simulink model "Ford_T3T6_ArchCnctnDigrm"  (R2016b)
settings: Solver=FixedStepDiscrete  StartTime=0.0  StopTime=10.0  RelTol=1e-3  EnableMultiTasking=on
libraries: canmsglib x15
(part 14 of 15)

== system Ford_T3T6_ArchCnctnDigrm/Ford CFs/FIH Read and Write/FIH write/CF055A_FordBlaBoxCanHiSpdWr1 ==
  EcuId : Inport
  FordEpsSysSt : Inport  Port=2
  FordVehBBMsgOutp1HiPart : Outport
  FordVehBBMsgOutp1LoPart : Outport  Port=2
  FordVehBBMsgOutp2HiPart : Outport  Port=3
  FordVehBBMsgOutp2LoPart : Outport  Port=4
  FordVehBBMsgOutp3HiPart : Outport  Port=5
  FordVehBBMsgOutp3LoPart : Outport  Port=6
  FordVehBBMsgOutp4HiPart : Outport  Port=7
  FordVehBBMsgOutp4LoPart : Outport  Port=8
  FordVehHitchToTrlrAxle : Outport  Port=9
  FordVehLaneAssiAvl : Outport  Port=10
  FordVehLaneAssiDeny : Outport  Port=11
  FordVehLaneAssiHandsOff : Outport  Port=12
  FordVehLatCtrlLimSts : Outport  Port=13
  FordVehLatCtrlSteerSts : Outport  Port=14
  FordVehLoSpdMtnCtrlBrkDecelEnaReq : Outport  Port=15
  FordVehLoSpdMtnCtrlBrkTqReq : Outport  Port=16
  FordVehTrfcJamAvdncHandsOnConf : Outport  Port=17
  FordVehTrlrAgMax : Outport  Port=18
  FordVehTrlrAgOffs : Outport  Port=19
  FordVehTrlrAgTarCalcn : Outport  Port=20
  FordVehTrlrAgWarn : Outport  Port=21
  FordVehTrlrAidEnaSts : Outport  Port=22
  FordVehTrlrAidMsgTxtReq : Outport  Port=23
  FordVehTrlrAidSetupSts : Outport  Port=24
  FordVehTrlrAidTarIdnReq : Outport  Port=25
  FordVehTrlrAidTrlredReq : Outport  Port=26
  FordVehTrlrHitchLampReq : Outport  Port=27
  FordVehVelMaxReqTrlrAid : Outport  Port=28
  FordVehVelTrlrAidReq : Outport  Port=29
  FIH_Write_FIH_Msg_1_High : Outport  Port=30
  FIH_Write_FIH_Msg_1_Low : Outport  Port=31
  FIH_Write_FIH_Msg_2_High : Outport  Port=32
  FIH_Write_FIH_Msg_2_Low : Outport  Port=33
  FIH_Write_FIH_Msg_3_High : Outport  Port=34
  FIH_Write_FIH_Msg_3_Low : Outport  Port=35
  FIH_Write_FIH_Msg_4_High : Outport  Port=36
  FIH_Write_FIH_Msg_4_Low : Outport  Port=37
  FIH_Write_LATCTL_HS_CAN : Outport  Port=38
  FIH_Write_LA_HS_CAN : Outport  Port=39
  FIH_Write_LsmcBrkDecel_Request : Outport  Port=40
  FIH_Write_TBA_to_EPAS_INFO : Outport  Port=41
  FIH_Write_TBA_to_LA_Data3 : Outport  Port=42
  FIH_Write_TBA_to_TrlrAid_Data2 : Outport  Port=43

== system Ford_T3T6_ArchCnctnDigrm/Ford CFs/FIH Read and Write/FIH write/CF058A_FordBlaBoxDiagcWr ==
  ActvNiblCmpIntSts : Outport
  LaneDprtrWarnIntSts : Outport  Port=2
  LaneKeepAssiIntSts : Outport  Port=3
  LatCtrlIntSts : Outport  Port=4
  PullDriftCmpIntSts : Outport  Port=5
  SrvPullDriftCmpAct : Outport  Port=6
  SrvPullDriftCmpRstVal : Outport  Port=7
  TrlrBackupAssiIntSts : Outport  Port=8
  FIH_Write_ANC_Int_Status_DID : Outport  Port=9
  FIH_Write_LATCTL_Int_Status_DID : Outport  Port=10
  FIH_Write_LDW_Int_Status_DID : Outport  Port=11
  FIH_Write_LKA_Int_Status_DID : Outport  Port=12
  FIH_Write_PDC_Actual_DID : Outport  Port=13
  FIH_Write_PDC_Int_Status_DID : Outport  Port=14
  FIH_Write_PDC_Service_DID : Outport  Port=15
  FIH_Write_TBA_Int_Status_DID : Outport  Port=16

== system Ford_T3T6_ArchCnctnDigrm/Ford CFs/FIH Read and Write/FIH write/CF060A_FordBlaBoxFeatStWr1 ==
  FordActvNiblCtrlFeatSt : Outport
  FordActvNiblCtrlSwVers : Outport  Port=2
  FordActvNiblCtrlTqReq : Outport  Port=3
  FordBlaBoxSwVers : Outport  Port=4
  FordLaneAssiSwVers : Outport  Port=5
  FordLaneDprtrWarnFeatSt : Outport  Port=6
  FordLaneDprtrWarnTqReq : Outport  Port=7
  FordLaneKeepAssiFeatSt : Outport  Port=8
  FordLaneKeepAssiTqReq : Outport  Port=9
  FordLatCtrlFeatSt : Outport  Port=10
  FordLatCtrlTqReq : Outport  Port=11
  FordPullDriftCmpFeatSt : Outport  Port=12
  FordPullDriftCmpLrngFeatSt : Outport  Port=13
  FordPullDriftCmpSwVers : Outport  Port=14
  FordPullDriftCmpTqReq : Outport  Port=15
  FordResrchFctSwVers : Outport  Port=16
  FordTrlrBackupAssiSwVers : Outport  Port=17
  FIH_Write_ANC_Arbiter : Outport  Port=18
  FIH_Write_ANC_SW_Version : Outport  Port=19
  FIH_Write_FIH_SW_Version : Outport  Port=20
  FIH_Write_LATCTL_Arbiter : Outport  Port=21
  FIH_Write_LA_SW_Version : Outport  Port=22
  FIH_Write_LDW_Arbiter : Outport  Port=23
  FIH_Write_LKA_Arbiter : Outport  Port=24
  FIH_Write_PDCLearning_Arbiter : Outport  Port=25
  FIH_Write_PDC_Arbiter : Outport  Port=26
  FIH_Write_PDC_SW_Version : Outport  Port=27
  FIH_Write_RF_SW_Version : Outport  Port=28
  FIH_Write_TBA_SW_Version : Outport  Port=29

== system Ford_T3T6_ArchCnctnDigrm/Ford CFs/FIH Read and Write/FIH write/CF090A_FordBlaBoxCanHiSpdWr2 ==
  EcuId : Inport
  FordEpsSysSt : Inport  Port=2
  FordVehEvasSteerAssiSts : Outport
  FIH_Write_ESA_HS_CAN : Outport  Port=2

== system Ford_T3T6_ArchCnctnDigrm/Ford CFs/FIH Read and Write/FIH write/CF091A_FordBlaBoxDiagcWr2 ==
  FordSteerTqDstbcRejctnIntSts : Outport
  FordEvasSteerAssiIntSts : Outport  Port=2
  FordTqSteerCmpActvnCntr : Outport  Port=3
  FordBrkPlsRednActvnCntr : Outport  Port=4
  FIH_Write_STDR_Int_Status_DID : Outport  Port=5
  FIH_Write_ESA_Int_Status_DID : Outport  Port=6
  FIH_Write_TSC_Activation_Cnt : Outport  Port=7
  FIH_Write_BPR_Activation_Cnt : Outport  Port=8

== system Ford_T3T6_ArchCnctnDigrm/Ford CFs/FIH Read and Write/FIH write/CF092A_FordBlaBoxFeatStWr2 ==
  FordSteerTqDstbcRejctnSwVers : Outport  OutMin=[0]  OutMax=[4294967295]  OutDataTypeStr=uint32  Unit=Uls
  FordEvasSteerAssiSwVers : Outport  Port=2  OutMin=[0]  OutMax=[4294967295]  OutDataTypeStr=uint32  Unit=Uls
  FordSteerDstbcRejctnFeatSt : Outport  Port=3  OutMin=[0]  OutMax=[255]  OutDataTypeStr=uint8  Unit=Cnt
  FordEvasSteerAssiFeatSt : Outport  Port=4  OutMin=[0]  OutMax=[255]  OutDataTypeStr=uint8  Unit=Cnt
  FordSteerTqDstbcRejctnTqReq : Outport  Port=5  OutMin=[-32]  OutMax=[31.99]  Unit=HwNwtMtr
  FordEvasSteerAssiTqReq : Outport  Port=6  OutMin=[-64]  OutMax=[63.99]  Unit=HwNwtMtr

== system Ford_T3T6_ArchCnctnDigrm/Ford CFs/FIH Read and Write/FIH write/CF094A_FordBlaBoxNvmWr1 ==
  EcuId : Inport
  FordBlaBoxLaneAssiByte : Outport
  FordBlaBoxPullDriftCmpByte : Outport  Port=2
  FordBlaBoxTrlrBackupByte : Outport  Port=3
  FIH_LA_Write_NV_Byte : Outport  Port=4
  FIH_PDC_Write_NV_Byte : Outport  Port=5
  FIH_TBA_Write_NV_Byte : Outport  Port=6

== system Ford_T3T6_ArchCnctnDigrm/Generate Steering Command/Openloop Steering Command/GenerateSteeringCommand/Assist ==
  note: NM001
  note: NM001
  note: Is being used by GM CF010C. Do we need in ford??
  note: ASIL D
  note: ASIL D
  note: ASIL B
  note: ASIL D Safety Mech
  note: ASIL D
  note: WIR Not being used
  note: WIR Not being used
  note: Is being used by GM CF010C. Do we need in ford??
  note: NM001
  HwTqSwp : Inport
  Ground{,1..3} (4 alike) : Ground
  SF001A_Assi : Subsystem  Tag=1.6.0  Description=The Assist Function applies an appropriate level of motor torque based on handwheel torque andvehicle speed. Its output is modified according to several inputs from other functions. Theseother factors may modify handwheel torque signal, provide blending to alternative calibration tables,or add/subtract values from the calculated assist value.
      settings: AttributesFormatString=Version: %<Tag>
  SF012A_HysCmp : Subsystem  Tag=1.2.1  Description=This function improves steering precision and feel by compensating for physical friction and efficiency losses. Due to the vibratory nature of a vehicle, the calibrations associated with these physical attributes are allowed to vary according to vehicle speed and the magnitude of Wheel Imbalance Rejection function command. The function includes a feature to deal with changing physical system properties over temperature operating range. It also incorporates calibration tables used to modify how the compensation is applied during transitions between operating quadrants and during periods of near-zero handwheel torque. Finally, the function may be disabled for purposes of bench testing.
      settings: AttributesFormatString=Version: %<Tag>
  SF028A_AssiHiFrq : Subsystem  Tag=1.2.1  Description=This function provides a means of compensating for system inertia and road feedback. It is tunable over both vehicle speed and handwheel torque to obtain the desired level of disturbance rejection under various operating conditions. It passes handwheel torque through a high-pass filter and multiplies the resulting signal by a tunable gain factor. The output is known as high-frequency assist and is simply added to the usual assist calculated elsewhere.
      settings: AttributesFormatString=Version: %<Tag>
  SF029A_StabyCmp : Subsystem  Tag=1.3.2  Description=This function provides in-vehicle stability of EPS behavior. To maximize steering feel, the function blends between two different tunings based on vehicle speed and low frequency handwheel torque. Because system gains may get multiplied by various scale factors, either from serial communications or from other software functions, this function provides a second blending feature. This model is designed using the best-known implementation at this time.
      settings: AttributesFormatString=Version: %<Tag>
  SF034B_AssiPahSum : Subsystem  Tag=1.0.1  Description=This function just merges command signals, and is used for vehicle programs that do not need the extra features of the SF034A firewall function.
      settings: AttributesFormatString=Version: %<Tag>
  AssiCmd : Outport
  AssiCmdBas : Outport  Port=2
  tag scope: AssiCmd=global, AssiCmdBas=global, AssiHiFrqCmd=global, HysCmpCmd=global
  wires:
  SF029A_StabyCmp/1(AssiCmd) -> [AssiCmd], AssiCmd/1
  [FltInj_f32] -> SF029A_StabyCmp/6(FltInj_f32)
  SF001A_Assi/1(AssiCmdBas) -> AssiCmdBas/1, SF034B_AssiPahSum/1(AssiCmdBas), [AssiCmdBas]
  SF028A_AssiHiFrq/1(AssiHiFrqCmd) -> SF034B_AssiPahSum/2(AssiHiFrqCmd), [AssiHiFrqCmd]
  [AssiCmdBasSca] -> SF029A_StabyCmp/1(AssiCmdBasSca)
  [VehSpd] -> SF029A_StabyCmp/5(VehSpd)
  SF034B_AssiPahSum/1(AssiCmdSum) -> SF029A_StabyCmp/2(AssiCmdSum)
  Ground/1 -> SF029A_StabyCmp/3(AssiPahLimrActv)
  [AssiCmdBas] -> SF012A_HysCmp/1(AssiCmdBas)
  [AssiMechT] -> SF012A_HysCmp/2(AssiMechT)
  [HwTq] -> SF012A_HysCmp/3(HwTq)
  [HysCmpCmdDi] -> SF012A_HysCmp/4(HysCmpCmdDi)
  [SysFricOffs] -> SF012A_HysCmp/5(SysFricOffs)
  [VehSpd] -> SF012A_HysCmp/6(VehSpd)
  [HwTqOvrl] -> SF012A_HysCmp/8(HwTqOvrl)
  [FltInj_f32] -> SF012A_HysCmp/9(FltInj_f32)
  SF012A_HysCmp/1(HysCmpCmd) -> [HysCmpCmd], SF034B_AssiPahSum/3(HysCmpCmd)
  Ground1/1 -> SF012A_HysCmp/7(WhlImbRejctnAmp)
  [AssiCmdBasSca] -> SF001A_Assi/1(AssiCmdBasSca)
  [AssiLnrGain] -> SF001A_Assi/2(AssiLnrGain)
  [AssiLnrGainEna] -> SF001A_Assi/3(AssiLnrGainEna)
  HwTqSwp/1 -> SF029A_StabyCmp/4(HwTq), SF028A_AssiHiFrq/1(HwTq), SF001A_Assi/4(HwTq)
  [HwTqHysOvrl] -> SF001A_Assi/5(HwTqHysOvrl)
  [HwTqOvrl] -> SF001A_Assi/6(HwTqOvrl)
  [ThermLimSlowFilMax] -> SF001A_Assi/7(ThermLimSlowFilMax)
  [VehSpd] -> SF001A_Assi/8(VehSpd)
  Ground3/1 -> SF001A_Assi/9(WhlImbRejctnAmp)
  [FltInj_f32] -> SF001A_Assi/10(FltInj_f32)
  [VehSpd] -> SF028A_AssiHiFrq/2(VehSpd)
  Ground2/1 -> SF028A_AssiHiFrq/3(WhlImbRejctnAmp)

== system Ford_T3T6_ArchCnctnDigrm/Generate Steering Command/Openloop Steering Command/GenerateSteeringCommand/Damping ==
  note: NM001
  note: NM001
  note: GM CF:CF025
      | Do we need it in Ford
  note: ASIL D
  note: ASIL D
  note: ASIL D
  note: CMS ?
  note: CMS?
  AssiCmdBas : Inport
  HwTqSwp : Inport  Port=2
  Ground : Ground
  SF003A_Dampg : Subsystem  Tag=1.5.0  Description=This function computes a motor damping torque derived primarily from handwheel velocity and scaled by other factors such as temperature and handwheel torque. Dampg shall be comprised of the sum of motor velocity damping and hydraulic power steering damping. Dampg shall be calibratable based on vehicle speed, handwheel torque, motor velocity, and assist.
      settings: AttributesFormatString=Version: %<Tag>
  SF014A_InertiaCmpVel : Subsystem  Tag=1.14.0  Description="Provide compensation that is dependent on filtering of motor velocity.  Primary purpose is to compensate for motor inertia at low frequencies (inertia compensation) and provide damping acting at higher frequencies (frequency dependent damping)."
      settings: AttributesFormatString=Version: %<Tag>
  SF035B_DampgPahSum : Subsystem  Tag=1.0.1  Description=This function is used for programs that do not need the extra features of the SF35A function.
      settings: AttributesFormatString=Version: %<Tag>
  DampgCmd : Outport
  tag scope: DampgCmdBas=global
  wires:
  SF003A_Dampg/1(DampgCmdBas) -> SF035B_DampgPahSum/1(DampgCmdBas), [DampgCmdBas]
  SF035B_DampgPahSum/1(DampgCmd) -> DampgCmd/1
  SF014A_InertiaCmpVel/1(InertiaCmpVelCmd) -> SF035B_DampgPahSum/2(InertiaCmpVelCmd)
  [InertiaCmpVelCmdDi] -> SF014A_InertiaCmpVel/4(InertiaCmpVelCmdDi)
  [FltInj_f32] -> SF014A_InertiaCmpVel/9(FltInj_f32)
  [VehLgtA] -> SF014A_InertiaCmpVel/6(VehLgtA)
  [InertiaCmpDecelGainDi] -> SF014A_InertiaCmpVel/3(InertiaCmpDecelGainDi)
  [MotVelCrf] -> SF014A_InertiaCmpVel/5(MotVelCrf)
  [VehSpd] -> SF014A_InertiaCmpVel/7(VehSpd)
  Ground/1 -> SF014A_InertiaCmpVel/8(WhlImbRejctnAmp)
  AssiCmdBas/1 -> SF003A_Dampg/1(AssiCmdBas), SF014A_InertiaCmpVel/1(AssiCmdBas)
  [AssiMechT] -> SF003A_Dampg/2(AssiMechT)
  [DampgCmdBasDi] -> SF003A_Dampg/3(DampgCmdBasDi)
  [DampgCmdOvrl] -> SF003A_Dampg/4(DampgCmdOvrl)
  [DampgCmdSca] -> SF003A_Dampg/5(DampgCmdSca)
  HwTqSwp/1 -> SF003A_Dampg/6(HwTq), SF014A_InertiaCmpVel/2(HwTq)
  [MotVelCrf] -> SF003A_Dampg/7(MotVelCrf)
  [VehSpd] -> SF003A_Dampg/8(VehSpd)
  [FltInj_f32] -> SF003A_Dampg/9(FltInj_f32)

== system Ford_T3T6_ArchCnctnDigrm/Generate Steering Command/Openloop Steering Command/GenerateSteeringCommand/Return ==
  note: ASIL B
  note: ASIL D
  note: CMS?
  note: CMS?
  note: CMS?
  note: CMS?
  note: CMS?
  note: NM001
  note: NM001
  note: NM001
  HwTqSwp : Inport
  SF002A_Rtn : Subsystem  Tag=2.3.0  Description="The Return function shall provide return to center capability to enhance vehicle returnability. This is achieved by applying output force toward center as a function of output position and vehicle speed Thisposition-based output is modified for the given driving situation basedon Handwheel  Torque, Handwheel Velocity, and system temperature.Outputcan be defeated or reduced until Handwheel Position is known with fullconfidence, which may occur at startup or upon completion of a learningprocedure. Finally, output is directly scaled higher or lower byadditional inputs (e.g. customer signals, diagnostics)."
      settings: AttributesFormatString=Version: %<Tag>
  SF036A_RtnPahFwl : Subsystem  Tag=1.2.0  Description=This function bounds motor torque commands from SF-02 Active Return, whose primary input is handwheel position. The incoming motor torque command is saturated to a set of upper and lower boundaries chosen according to handwheel position.
      settings: AttributesFormatString=Version: %<Tag>
  RtnCmd : Outport
  tag scope: RtnCmd=global, RtnCmdLimd=global
  wires:
  SF036A_RtnPahFwl/1(RtnCmdLimd) -> RtnCmd/1, [RtnCmdLimd]
  [AssiMechT] -> SF002A_Rtn/1(AssiMechT)
  [HwAg] -> SF002A_Rtn/2(HwAg)
  [HwAgAuthySca] -> SF002A_Rtn/3(HwAgAuthySca)
  [HwAgRtnOffs] -> SF002A_Rtn/4(HwAgRtnOffs)
  HwTqSwp/1 -> SF002A_Rtn/5(HwTq)
  [HwVel] -> SF002A_Rtn/6(HwVel)
  [RtnCmdDi] -> SF002A_Rtn/7(RtnCmdDi)
  [RtnCmdDiagcDi] -> SF002A_Rtn/8(RtnCmdDiagcDi)
  [RtnCmdSca] -> SF002A_Rtn/9(RtnCmdSca)
  [RtnCmdScaServo] -> SF002A_Rtn/10(RtnCmdScaServo)
  [VehSpd] -> SF002A_Rtn/11(VehSpd)
  [VehSpdVld] -> SF002A_Rtn/12(VehSpdVld)
  [FltInj_f32] -> SF002A_Rtn/13(FltInj_f32)
  [HwAg] -> SF036A_RtnPahFwl/1(HwAg)
  [MfgEnaSt] -> SF036A_RtnPahFwl/2(MfgEnaSt)
  SF002A_Rtn/1(RtnCmd) -> [RtnCmd]
  [RtnCmdDi] -> SF036A_RtnPahFwl/4(RtnCmdDi)
  [VehSpd] -> SF036A_RtnPahFwl/5(VehSpd)
  [SetNtcSts10] -> SF036A_RtnPahFwl/6(SetNtcSts)
  [RtnCmd] -> SF036A_RtnPahFwl/3(RtnCmd)

== system Ford_T3T6_ArchCnctnDigrm/Generate Steering Command/Openloop Steering Command/GenerateSteeringCommand/SF004B_AssiSumLim ==
  AssiCmd : Inport
  DampgCmd : Inport  Port=2
  EotActvCmd : Inport  Port=3
  EotAssiSca : Inport  Port=4
  EotDampgCmd : Inport  Port=5
  EotMotTqLim : Inport  Port=6
  HwTqLoaMtgtnEna : Inport  Port=7
  MotTqCmdLimDi : Inport  Port=8
  MotTqCmdOvrl : Inport  Port=9
  MotVelMrf : Inport  Port=10
  PinionCentrLrnCmd : Inport  Port=11
  PinionCentrLrnEna : Inport  Port=12
  PullCmpCmd : Inport  Port=13
  PwrLimrRednFac : Inport  Port=14
  RtnCmd : Inport  Port=15
  StallMotTqLim : Inport  Port=16
  SysMotTqCmdSca : Inport  Port=17
  ThermMotTqLim : Inport  Port=18
  ThermRednFac : Inport  Port=19
  TqLoaCmd : Inport  Port=20
  TqSteerMtgtnCmd : Inport  Port=21
  VehSpd : Inport  Port=22
  VehSpdMotTqLim : Inport  Port=23
  WhlImbRejctnCmd : Inport  Port=24
  GetNtcQlfrSts : Inport  Port=25
  SetNtcSts : Inport  Port=26
  MotTqCmd : Outport
  MotTqCmdLimdPreStall : Outport  Port=2
  MotTqCmdLimrMin : Outport  Port=3
  MotTqCmdPreLim : Outport  Port=4
  SysProtnRednFac : Outport  Port=5
  SetManTqCmd : Outport  Port=6

== system Ford_T3T6_ArchCnctnDigrm/Generate Steering Command/Openloop Steering Command/GenerateSteeringCommand/SF020B_PosnTrakgServo ==
  HwAg : Inport
  HwTq : Inport  Port=2
  MotVelCrf : Inport  Port=3
  PosnServoEna : Inport  Port=4
  PosnServoHwAg : Inport  Port=5
  PosnServoHwVel : Inport  Port=6
  PosnServoIntgtrOffs : Inport  Port=7
  PosnTrakgArbnFltMtgtnEna : Inport  Port=8
  VehSpd : Inport  Port=9
  PosnServoCmd : Outport
  PosnServoIntgtrSt : Outport  Port=2

== system Ford_T3T6_ArchCnctnDigrm/Generate Steering Command/Openloop Steering Command/System Protection/EoTProtection ==
  note: ASIL B
  note: ASIL B
  note: ASIL D
  note: NM001
  note: NM001
  note: NM001
  SF016A_VehSpdLimr : Subsystem  Tag=2.0.1  Description=The Vehicle Speed Limiting Function determines a limited assist torque command value as a function of vehicle speed and handwheel position to manage mechanical fatigue near end-of-travel positions.
      settings: AttributesFormatString=Version: %<Tag>
  SF018A_EotProtn : Subsystem  Tag=1.11.0  Description=The End of Travel Protection function specifies performance attributes as the steering system approaches the mechanical end of travel of the steering gear. There are three primary functions: Velocity Impact (VI), Soft Stops (SS), and Software Rack Limiter (SRL). The purpose of VI is to limit the assist for high steering velocity. The purpose of SS is to scale down the assist and provide damping. The SRL is intended to simulate a hardware rack limiter.
      settings: AttributesFormatString=Version: %<Tag>
  SF027A_EotProtnFwl : Subsystem  Tag=1.3.1  Description="This function applies boundary limitations on motor torque commands from SF018A (EOT Protection)including the EOTDamping and EOTActive.   The motor torque commands are saturation limited toupper and lower boundaries.  Three criteria are tested to determine the firewall limit to be applied:1) Determine if a command is within a statically dterined intended active range for the EOT Protectionfunction.  This contrasts with the dynamically determined active range for SF018 based on the learnedend of travel limits.  If determined to be within the active range then apply an upper and lower boundary.2) If Handwheel Position is inboard of the active region (eg between +/- X0) then apply simple saturationlimit preventing a large command from being output.3) If Handwheel Authority is below a  calibration threshold value, then apply a simple saturation limitpreventing a large command from being output."
      settings: AttributesFormatString=Version: %<Tag>
  EotActvCmd : Outport
  EotDampgCmd : Outport  Port=2
  EotAssiSca : Outport  Port=3
  EotMotTqLim : Outport  Port=4
  VehSpdMotTqLim : Outport  Port=5
  tag scope: EotActvCmd=global, EotAssiSca=global, EotDampgCmd=global, EotMotTqLim=global
  wires:
  SF018A_EotProtn/2(EotAssiSca) -> EotAssiSca/1, [EotAssiSca]
  SF018A_EotProtn/4(EotMotTqLim) -> EotMotTqLim/1, [EotMotTqLim]
  [HwAg] -> SF016A_VehSpdLimr/1(HwAg)
  [PinionAgConf] -> SF016A_VehSpdLimr/2(HwAgAuthy)
  [HwAgEotCcw] -> SF016A_VehSpdLimr/3(HwAgEotCcw)
  [HwAgEotCw] -> SF016A_VehSpdLimr/4(HwAgEotCw)
  [VehSpd] -> SF016A_VehSpdLimr/5(VehSpd)
  SF016A_VehSpdLimr/1(VehSpdMotTqLim) -> VehSpdMotTqLim/1
  [EotProtnDi] -> SF027A_EotProtnFwl/3(EotProtnDi)
  [HwAg] -> SF027A_EotProtnFwl/4(HwAg)
  [MfgEnaSt] -> SF027A_EotProtnFwl/5(MfgEnaSt)
  [MotVelCrf] -> SF027A_EotProtnFwl/6(MotVelCrf)
  [PinionAgConf] -> SF027A_EotProtnFwl/7(PinionAgConf)
  [VehSpd] -> SF027A_EotProtnFwl/8(VehSpd)
  [SetNtcSts] -> SF027A_EotProtnFwl/9(SetNtcSts)
  SF018A_EotProtn/1(EotActvCmd) -> SF027A_EotProtnFwl/1(EotActvCmd), [EotActvCmd]
  SF018A_EotProtn/3(EotDampgCmd) -> SF027A_EotProtnFwl/2(EotDampgCmd), [EotDampgCmd]
  SF027A_EotProtnFwl/1(EotActvCmdLimd) -> EotActvCmd/1
  SF027A_EotProtnFwl/2(EotDampgCmdLimd) -> EotDampgCmd/1
  [EotProtnDi] -> SF018A_EotProtn/1(EotProtnDi)
  [HwAg] -> SF018A_EotProtn/2(HwAg)
  [PinionAgConf] -> SF018A_EotProtn/3(HwAgAuthy)
  [HwAgCcwDetd] -> SF018A_EotProtn/4(HwAgCcwDetd)
  [HwAgCwDetd] -> SF018A_EotProtn/5(HwAgCwDetd)
  [HwAgEotCcw] -> SF018A_EotProtn/6(HwAgEotCcw)
  [HwAgEotCw] -> SF018A_EotProtn/7(HwAgEotCw)
  [HwTq] -> SF018A_EotProtn/8(HwTq)
  [MotVelCrf] -> SF018A_EotProtn/9(MotVelCrf)
  [SysMotTqCmdSca] -> SF018A_EotProtn/10(SysMotTqCmdSca)
  [VehSpd] -> SF018A_EotProtn/11(VehSpd)

== system Ford_T3T6_ArchCnctnDigrm/Generate Steering Command/Openloop Steering Command/System Protection/Motor Protection ==
  note: Which MM??
  note: ASIL B
  note: ASIL B
  note: Which MM??
  note: NM001
  note: NM001
  MotTqCmdLimdPreStall : Inport
  SF009A_DutyCycThermProtn : Subsystem  Tag=4.0.0  Description=The purpose of the Thermal Duty Cycle Protection is to limitand protect the system from excessive use, based on motor rotational velocity and system temperature.It also provides protection status information for use by other functions.
      settings: AttributesFormatString=Version: %<Tag>
  SF017A_HiLoadStallLimr : Subsystem  Tag=3.0.0  Description="This function protects the system from prolonged intervals of high assist torque at near-stall conditions.  In other words, it quickly limits large torque commands if the motor velocity is below a calibratable threshold. The High Load Stall Limiter function uses a low-pass filter (LPF) and a torque limit table to reduce the maximum allowed torque command under certain operating conditions.  When motor velocity is equal to or falls below the calibratable threshold, the torque command is applied to the input of the low-pass filter.  The output of the filter ramps up and indexes into the torque limit table.  The output of this table is the maximum allowed torque command.  A slew limit calibration governs the transition rate of the table output."
      settings: AttributesFormatString=Version: %<Tag>
  StallMotTqLim : Outport
  ThermMotTqLim : Outport  Port=2
  tag scope: DutyCycThermProtnMaxOutp=global, StallMotTqLim=global, ThermDutyCycProtnLoadDptLim=global, ThermDutyCycProtnTDptLim=global, ThermLimSlowFilMax=global, ThermMotTqLim=global, ThermRednFac=global
  wires:
  SF009A_DutyCycThermProtn/5(ThermMotTqLim) -> ThermMotTqLim/1, [ThermMotTqLim]
  [DualEcuFltMtgtnEna] -> SF017A_HiLoadStallLimr/1(DualEcuFltMtgtnEna)
  [MotAndThermProtnLoaMod] -> SF017A_HiLoadStallLimr/2(MotAndThermProtnLoaMod)
  MotTqCmdLimdPreStall/1 -> SF017A_HiLoadStallLimr/3(MotTqCmdLimdPreStall)
  [MotVelCrf] -> SF017A_HiLoadStallLimr/4(MotVelCrf)
  [StallMotTqLimDi] -> SF017A_HiLoadStallLimr/5(StallMotTqLimDi)
  SF017A_HiLoadStallLimr/1(StallMotTqLim) -> StallMotTqLim/1, [StallMotTqLim]
  [DiagcStsLimdTPrfmnc] -> SF009A_DutyCycThermProtn/1(DiagcStsLimdTPrfmnc)
  [DualEcuFltMtgtnEna] -> SF009A_DutyCycThermProtn/2(DualEcuFltMtgtnEna)
  [DutyCycThermProtnDi] -> SF009A_DutyCycThermProtn/3(DutyCycThermProtnDi)
  [EcuTFild] -> SF009A_DutyCycThermProtn/4(EcuTFild)
  [IgnTiOff] -> SF009A_DutyCycThermProtn/5(IgnTiOff)
  [MotAndThermProtnLoaMod] -> SF009A_DutyCycThermProtn/6(MotAndThermProtnLoaMod)
  [MotCurrPeakEstimd] -> SF009A_DutyCycThermProtn/7(MotCurrPeakEstimd)
  [MotCurrPeakEstimdFild] -> SF009A_DutyCycThermProtn/8(MotCurrPeakEstimdFild)
  [MotFetT] -> SF009A_DutyCycThermProtn/9(MotFetT)
  [MotMagT] -> SF009A_DutyCycThermProtn/10(MotMagT)
  [MotVelCrf] -> SF009A_DutyCycThermProtn/11(MotVelCrf)
  [MotWidgT] -> SF009A_DutyCycThermProtn/12(MotWidgT)
  [VehTiVld] -> SF009A_DutyCycThermProtn/13(VehTiVld)
  [NvMProxy_GetErrorStatus] -> SF009A_DutyCycThermProtn/14(FilStVal_GetErrorStatus)
  [NvMProxy_SetRamBlockStatus] -> SF009A_DutyCycThermProtn/15(FilStVal_SetRamBlockStatus)
  [SetNtcSts8] -> SF009A_DutyCycThermProtn/16(SetNtcSts)
  SF009A_DutyCycThermProtn/1(DutyCycThermProtnMaxOutp) -> [DutyCycThermProtnMaxOutp]
  SF009A_DutyCycThermProtn/2(ThermDutyCycProtnLoadDptLim) -> [ThermDutyCycProtnLoadDptLim]
  SF009A_DutyCycThermProtn/3(ThermDutyCycProtnTDptLim) -> [ThermDutyCycProtnTDptLim]
  SF009A_DutyCycThermProtn/4(ThermLimSlowFilMax) -> [ThermLimSlowFilMax]
  SF009A_DutyCycThermProtn/6(ThermRednFac) -> [ThermRednFac]

== system Ford_T3T6_ArchCnctnDigrm/Generate Steering Command/Openloop Steering Command/System Protection/SF038A_LimrCdng ==
  EotAssiSca : Inport
  EotMotTqLim : Inport  Port=2
  StallMotTqLim : Inport  Port=3
  SysMotTqCmdSca : Inport  Port=4
  ThermMotTqLim : Inport  Port=5
  VehSpd : Inport  Port=6
  VehSpdMotTqLim : Inport  Port=7
  FltInj_f32 : Inport  Port=8
  EotAssiScaCdnd : Outport
  EotMotTqLimCdnd : Outport  Port=2
  StallMotTqLimCdnd : Outport  Port=3
  SysMotTqCmdScaCdnd : Outport  Port=4
  ThermMotTqLimCdnd : Outport  Port=5
  VehSpdMotTqLimCdnd : Outport  Port=6

== system Ford_T3T6_ArchCnctnDigrm/Monitor System/Inferred Signals/HwAg before IMC/CF075A_FordHwAgArbn ==
  FordVehSteerPinionAgOffs : Inport
  FordVehSteerPinionOffsSts : Inport  Port=2
  FordVehSteerPinionOffsChks : Inport  Port=3
  FordVehSteerPinionOffsCnt : Inport  Port=4
  HwAgFinal : Inport  Port=5
  HwAgNotCorrd : Inport  Port=6
  PinionVel : Inport  Port=7
  PinionVelConf : Inport  Port=8
  FordAbsPrsnt : Inport  Port=9
  FordSteerAgClrFlg : Inport  Port=10
  HwAgIdptSig : Inport  Port=11
  GetRefTmr100MicroSec32bit : Inport  Port=12
  GetTiSpan100MicroSec32bit : Inport  Port=13
  NonAbsOffsVldFlg_GetErrorStatus : Inport  Port=14
  NonAbsOffsVldFlg_SetRamBlockStatus : Inport  Port=15
  NonAbsOffs_GetErrorStatus : Inport  Port=16
  NonAbsOffs_SetRamBlockStatus : Inport  Port=17
  PrevIgnCycVal_GetErrorStatus : Inport  Port=18
  PrevIgnCycVal_SetRamBlockStatus : Inport  Port=19
  SetNtcSts : Inport  Port=20
  FordCmpdHwPosn : Outport
  FordCmpdHwPosnQlyFac : Outport  Port=2
  FordHwVel : Outport  Port=3
  FordHwVelVld : Outport  Port=4
  FordPosnOffsVld : Outport  Port=5
  FordRelHwPosn : Outport  Port=6
  FordRelHwPosnVld : Outport  Port=7

== system Ford_T3T6_ArchCnctnDigrm/Monitor System/Inferred Signals/HwAg before IMC/SF041A_CmplncErr ==
  HwTq : Inport
  MotTqCmdCrf : Inport  Port=2
  CmplncErrMotToPinion : Outport
  CmplncErrPinionToHw : Outport  Port=2

== system Ford_T3T6_ArchCnctnDigrm/Monitor System/Inferred Signals/HwAg before IMC/SF042A_HwAgSnsrls ==
  CmplncErrMotToPinion : Inport
  HwTq : Inport  Port=2
  MotAgCumvAlgndCrf : Inport  Port=3
  MotAgCumvAlgndVld : Inport  Port=4
  MotAgMeclIdptSig : Inport  Port=5
  MotTqCmdCrf : Inport  Port=6
  MotVelCrf : Inport  Port=7
  PinionAg : Inport  Port=8
  PinionAgConf : Inport  Port=9
  VehSpd : Inport  Port=10
  VehSpdVld : Inport  Port=11
  VehYawRate : Inport  Port=12
  VehYawRateVld : Inport  Port=13
  WhlFrqVld : Inport  Port=14
  WhlLeFrq : Inport  Port=15
  WhlRiFrq : Inport  Port=16
  GetNtcQlfrSts : Inport  Port=17
  GetRefTmr100MicroSec32bit : Inport  Port=18
  GetTiSpan100MicroSec32bit : Inport  Port=19
  StordLstPrm_SetRamBlockStatus : Inport  Port=20
  HwAgSnsrls : Outport
  HwAgSnsrlsConf : Outport  Port=2
  FSnsrlsHwCentr : Outport  Port=3
  RstSnsrlsHwCentr : Outport  Port=4

== system Ford_T3T6_ArchCnctnDigrm/Monitor System/Inferred Signals/HwAg before IMC/SF045A_HwAgSysArbn ==
  CmplncErrPinionToHw : Inport
  HwAg : Inport  Port=2
  HwAgCorrd : Inport  Port=3
  HwAgIdptSig : Inport  Port=4
  HwAgSnsrls : Inport  Port=5
  HwAgSnsrlsConf : Inport  Port=6
  HwTq : Inport  Port=7
  MotVelCrf : Inport  Port=8
  MotVelVld : Inport  Port=9
  GetNtcQlfrSts : Inport  Port=10
  FltInj_f32 : Inport  Port=11
  GetRefTmr100MicroSec32bit : Inport  Port=12
  GetTiSpan100MicroSec32bit : Inport  Port=13
  SetNtcSts : Inport  Port=14
  HwAgFinal : Outport
  HwAgNotCorrd : Outport  Port=2
  HwAgToSerlCom : Outport  Port=3
  HwAgVldToSerlCom : Outport  Port=4
  HwVel : Outport  Port=5
  HwVelToSerlCom : Outport  Port=6
  PinionAg : Outport  Port=7
  PinionAgConf : Outport  Port=8
  PinionVel : Outport  Port=9
  PinionVelConf : Outport  Port=10

== system Ford_T3T6_ArchCnctnDigrm/Monitor System/Measured Signals/ADC/CM012A_FordT3McuCfg ==
  Adc0Faild : Inport
  Adc1Faild : Inport  Port=2
  Adc1RawRes : Inport  Port=3
  EcuId : Inport  Port=4
  MotCtrlAdc0RawRes : Inport  Port=5
  GetRefTmr1MicroSec32bit : Inport  Port=6
  GetTiSpan1MicroSec32bit : Inport  Port=7
  Adc1ScanGroup2Ref0 : Outport
  Adc1ScanGroup2Ref1 : Outport  Port=2
  Adc1ScanGroup3Ref0 : Outport  Port=3
  Adc1ScanGroup3Ref1 : Outport  Port=4
  Adc1SelfDiag0 : Outport  Port=5
  Adc1SelfDiag2 : Outport  Port=6
  Adc1SelfDiag4 : Outport  Port=7
  BattRtnCurrAdc : Outport  Port=8
  BattRtnCurrAdcFaild : Outport  Port=9
  BattVltg : Outport  Port=10
  BattVltgAdcFaild : Outport  Port=11
  BattVltgSwd1 : Outport  Port=12
  BattVltgSwd1AdcFaild : Outport  Port=13
  ChrgPmpDiag : Outport  Port=14
  ChrgPmpDiagAdcFaild : Outport  Port=15
  EcuT : Outport  Port=16
  EcuTAdcFaild : Outport  Port=17
  HwAg1SnsrNr : Outport  Port=18
  HwAg1SnsrTyp : Outport  Port=19
  MotAg2Cos : Outport  Port=20
  MotAg2CosAdcFaild : Outport  Port=21
  MotAg2Sin : Outport  Port=22
  MotAg2SinAdcFaild : Outport  Port=23
  MotAg5CosAdcFaild : Outport  Port=24
  MotAg5SinAdcFaild : Outport  Port=25
  MotAg6CosAdcFaild : Outport  Port=26
  MotAg6SinAdcFaild : Outport  Port=27
  MotCurrAdcPeakAAdcFaild : Outport  Port=28
  MotCurrAdcPeakBAdcFaild : Outport  Port=29
  MotCurrAdcPeakCAdcFaild : Outport  Port=30
  MotCurrAdcVlyAAdcFaild : Outport  Port=31
  MotCurrAdcVlyBAdcFaild : Outport  Port=32
  MotCurrAdcVlyCAdcFaild : Outport  Port=33
  MotCurrSnsrOffs1AdcFaild : Outport  Port=34
  PwrDiscnctSwtDiag : Outport  Port=35
  PwrDiscnctSwtDiagAdcFaild : Outport  Port=36
  MotDrvr1IninTestCmpl : Outport  Port=37
  MotCtrlAdc0ScanGroup2Ref0 : Outport  Port=38
  MotCtrlAdc0ScanGroup2Ref1 : Outport  Port=39
  MotCtrlAdc0ScanGroup3Ref0 : Outport  Port=40
  MotCtrlAdc0ScanGroup3Ref1 : Outport  Port=41
  MotCtrlAdc0SelfDiag0 : Outport  Port=42
  MotCtrlAdc0SelfDiag2 : Outport  Port=43
  MotCtrlAdc0SelfDiag4 : Outport  Port=44
  MotCtrlMotAg5Cos : Outport  Port=45
  MotCtrlMotAg5Sin : Outport  Port=46
  MotCtrlMotAg6Cos : Outport  Port=47
  MotCtrlMotAg6Sin : Outport  Port=48
  MotCtrlMotCurrAdcPeakA : Outport  Port=49
  MotCtrlMotCurrAdcPeakB : Outport  Port=50
  MotCtrlMotCurrAdcPeakC : Outport  Port=51
  MotCtrlMotCurrAdcVlyA : Outport  Port=52
  MotCtrlMotCurrAdcVlyB : Outport  Port=53
  MotCtrlMotCurrAdcVlyC : Outport  Port=54
  MotCtrlMotCurrSnsrOffs1 : Outport  Port=55

== system Ford_T3T6_ArchCnctnDigrm/Monitor System/Measured Signals/ADC/ES251A_BattRtnCurr ==
  BattRtnCurrAdc : Inport  OutMin=[0]  OutMax=[5]  OutDataTypeStr=single  Unit=Volt
  BattRtnCurrAdcFaild : Inport  Port=2  OutMin=[0]  OutMax=[1]  OutDataTypeStr=boolean  Unit=Cnt
  SplyCurrEstim : Inport  Port=3  OutMin=[-200]  OutMax=[200]  OutDataTypeStr=single  Unit=Ampr
  SysSt : Inport  Port=4  OutMin=[0]  OutMax=[3]  Unit=Cnt
  MotCtrlBattRtnCurrAdc : Inport  Port=5  OutMin=[0]  OutMax=[5]  OutDataTypeStr=single  Unit=Volt
  CnvSnpshtData_f32 : Inport  Port=6  OutMin=[[]]  OutMax=[[]]
  CnvSnpshtData_u08 : Inport  Port=7  OutMin=[[]]  OutMax=[[]]
  GetNtcQlfrSts : Inport  Port=8  OutMin=[0]  OutMax=[1]
  SetNtcStsAndSnpshtData : Inport  Port=9  OutMin=[0]  OutMax=[1]
  BattRtnCurrAmpr : Outport  OutMin=[-300]  OutMax=[300]  OutDataTypeStr=single  Unit=Ampr
  BattRtnCurrStsQlfr : Outport  Port=2  OutMin=[0]  OutMax=[2]  Unit=Cnt
  MotCtrlBattRtnCurrAmprFastLoop : Outport  Port=3  OutMin=[-300]  OutMax=[300]  OutDataTypeStr=single  Unit=Ampr

== system Ford_T3T6_ArchCnctnDigrm/Monitor System/Measured Signals/BatteryVoltage/ES250B_BattVltg ==
  BattSwdVltgCorrlnSts : Inport
  BattVltg : Inport  Port=2
  BattVltgSwd1 : Inport  Port=3
  BrdgVltg : Outport

== system Ford_T3T6_ArchCnctnDigrm/Monitor System/Measured Signals/BatteryVoltage/ES259B_BattVltgCorrln ==
  BattVltg : Inport
  BattVltgAdcFaild : Inport  Port=2
  BattVltgSwd1 : Inport  Port=3
  BattVltgSwd1AdcFaild : Inport  Port=4
  DiagcStsIvtr1Inactv : Inport  Port=5
  InhbBattVltgDiagc : Inport  Port=6
  StrtUpSt : Inport  Port=7
  SysSt : Inport  Port=8
  GetNtcQlfrSts : Inport  Port=9
  SetNtcSts : Inport  Port=10
  BattSwdVltgCorrlnSts : Outport
  BattVltgCorrlnIdptSig : Outport  Port=2
  DftBrdgVltgActv : Outport  Port=3
  SwdVltgLimd : Outport  Port=4

== system Ford_T3T6_ArchCnctnDigrm/Monitor System/Measured Signals/EcuTemp/ES210A_EcuTMeas ==
  EcuT : Inport
  EcuTAdcFaild : Inport  Port=2
  CnvSnpshtData_f32 : Inport  Port=3
  CnvSnpshtData_logl : Inport  Port=4
  GetNtcActv : Inport  Port=5
  SetNtcStsAndSnpshtData : Inport  Port=6
  DiagcStsLimdTPrfmnc : Outport
  EcuTFild : Outport  Port=2

== system Ford_T3T6_ArchCnctnDigrm/Monitor System/Measured Signals/HwAg Signal Measurement and  Arbitration/CM670A_HwAg1Meas ==
  HwAg1Polarity : Inport
  HwAg1SnsrTyp : Inport  Port=2
  CnvSnpshtData_f32 : Inport  Port=3
  CnvSnpshtData_u08 : Inport  Port=4
  FltInj_u08 : Inport  Port=5
  GetNtcQlfrSts : Inport  Port=6
  GetRefTmr1MicroSec32bit : Inport  Port=7
  GetTiSpan1MicroSec32bit : Inport  Port=8
  HwAg1IfFltLtch_GetErrorStatus : Inport  Port=9
  HwAg1IfFltLtch_SetRamBlockStatus : Inport  Port=10
  HwAg1Offs_GetErrorStatus : Inport  Port=11
  HwAg1Offs_SetRamBlockStatus : Inport  Port=12
  IoHwAb_SetFctPrphlHwAg1 : Inport  Port=13
  SetNtcStsAndSnpshtData : Inport  Port=14
  HwAg1 : Outport
  HwAg1Qlfr : Outport  Port=2
  HwAg1RollgCntr : Outport  Port=3
  HwAg1AutTrim : Outport  Port=4
  HwAg1ClrLtch : Outport  Port=5
  HwAg1ClrTrim : Outport  Port=6
  HwAg1ReadTrim : Outport  Port=7
  HwAg1TrimPrfmdSts : Outport  Port=8
  HwAg1WrTrim : Outport  Port=9

== system Ford_T3T6_ArchCnctnDigrm/Monitor System/Measured Signals/HwAg Signal Measurement and  Arbitration/ES238A_HwAgArbn ==
  HwAg1SnsrNr : Inport  OutMin=[0]  OutMax=[2]  OutDataTypeStr=uint8  Unit=Cnt
  HwAgA : Inport  Port=2  OutMin=[-900]  OutMax=[900]  OutDataTypeStr=single  Unit=HwDeg
  HwAgAQlfr : Inport  Port=3  OutMin=[0]  OutMax=[2]  OutDataTypeStr=Enum: SigQlfr1  Unit=Cnt
  HwAgARollgCntr : Inport  Port=4  OutMin=[0]  OutMax=[255]  OutDataTypeStr=uint8  Unit=Cnt
  HwAgB : Inport  Port=5  OutMin=[-900]  OutMax=[900]  OutDataTypeStr=single  Unit=HwDeg
  HwAgBQlfr : Inport  Port=6  OutMin=[0]  OutMax=[2]  OutDataTypeStr=Enum: SigQlfr1  Unit=Cnt
  HwAgBRollgCntr : Inport  Port=7  OutMin=[0]  OutMax=[255]  OutDataTypeStr=uint8  Unit=Cnt
  HwAgCorrlnSt : Inport  Port=8  OutMin=[0]  OutMax=[3]  OutDataTypeStr=uint8  Unit=Cnt
  FltInj_f32 : Inport  Port=9  OutMin=[[]]  OutMax=[[]]
  HwAg : Outport  OutMin=[-900]  OutMax=[900]  OutDataTypeStr=single  Unit=HwDeg

== system Ford_T3T6_ArchCnctnDigrm/Monitor System/Measured Signals/HwAg Signal Measurement and  Arbitration/ES239A_HwAgCorrln ==
  HwAg1SnsrNr : Inport  OutMin=[0]  OutMax=[2]  OutDataTypeStr=uint8  Unit=Cnt
  HwAgA : Inport  Port=2  OutMin=[-900]  OutMax=[900]  OutDataTypeStr=single  Unit=HwDeg
  HwAgAQlfr : Inport  Port=3  OutMin=[0]  OutMax=[2]  OutDataTypeStr=Enum: SigQlfr1  Unit=Cnt
  HwAgARollgCntr : Inport  Port=4  OutMin=[0]  OutMax=[255]  OutDataTypeStr=uint8  Unit=Cnt
  HwAgB : Inport  Port=5  OutMin=[-900]  OutMax=[900]  OutDataTypeStr=single  Unit=HwDeg
  HwAgBQlfr : Inport  Port=6  OutMin=[0]  OutMax=[2]  OutDataTypeStr=Enum: SigQlfr1  Unit=Cnt
  HwAgBRollgCntr : Inport  Port=7  OutMin=[0]  OutMax=[255]  OutDataTypeStr=uint8  Unit=Cnt
  FltInj_u08 : Inport  Port=8  OutMin=[[]]  OutMax=[[]]
  GetNtcQlfrSts : Inport  Port=9  OutMin=[0]  OutMax=[1]
  SetNtcSts : Inport  Port=10  OutMin=[0]  OutMax=[1]
  HwAgCorrlnSt : Outport  OutMin=[0]  OutMax=[3]  OutDataTypeStr=uint8  Unit=Cnt
  HwAgIdptSig : Outport  Port=2  OutMin=[0]  OutMax=[2]  OutDataTypeStr=uint8  Unit=Cnt

== system Ford_T3T6_ArchCnctnDigrm/Monitor System/Measured Signals/MotorAngle/ES241A_MotAg2Meas ==
  MotAg2Cos : Inport
  MotAg2CosAdcFaild : Inport  Port=2
  MotAg2Sin : Inport  Port=3
  MotAg2SinAdcFaild : Inport  Port=4
  MotAgMecl2Polarity : Inport  Port=5
  FltInj_f32 : Inport  Port=6
  GetNtcQlfrSts : Inport  Port=7
  MotAg2EolPrm_GetErrorStatus : Inport  Port=8
  MotAg2EolPrm_SetRamBlockStatus : Inport  Port=9
  SetNtcSts : Inport  Port=10
  MotAg2Mecl : Outport
  MotAg2MeclQlfr : Outport  Port=2
  MotAg2MeclRollgCntr : Outport  Port=3
  MotAg2VltgSqd : Outport  Port=4
  MotAg2MeasEolPrmRead : Outport  Port=5
  MotAg2MeasEolPrmWr : Outport  Port=6

== system Ford_T3T6_ArchCnctnDigrm/Monitor System/Measured Signals/MotorAngle/ES242A_MotAg5Meas ==
  MotAg5Cos : Inport
  MotAg5CosAdcFaild : Inport  Port=2
  MotAg5RawMecl : Inport  Port=3
  MotAg5Sin : Inport  Port=4
  MotAg5SinAdcFaild : Inport  Port=5
  MotVelMrf : Inport  Port=6
  MotCtrlMotAg5Cos : Inport  Port=7
  MotCtrlMotAg5CosRtAmpRecpr : Inport  Port=8
  MotCtrlMotAg5CosRtOffs : Inport  Port=9
  MotCtrlMotAg5Polarity : Inport  Port=10
  MotCtrlMotAg5Sin : Inport  Port=11
  MotCtrlMotAg5SinRtAmpRecpr : Inport  Port=12
  MotCtrlMotAg5SinRtOffs : Inport  Port=13
  CnvSnpshtData_f32 : Inport  Port=14
  CnvSnpshtData_logl : Inport  Port=15
  GetNtcQlfrSts : Inport  Port=16
  GetRefTmr1MicroSec32bit : Inport  Port=17
  MotAg5EolPrm_GetErrorStatus : Inport  Port=18
  MotAg5EolPrm_SetRamBlockStatus : Inport  Port=19
  MotAg5StVari_GetErrorStatus : Inport  Port=20
  MotAg5StVari_SetRamBlockStatus : Inport  Port=21
  SetNtcStsAndSnpshtData : Inport  Port=22
  MotAg5CosRtAmpRecpr : Outport
  MotAg5CosRtOffs : Outport  Port=2
  MotAg5MeclQlfr : Outport  Port=3
  MotAg5MeclRollgCntr : Outport  Port=4
  MotAg5SinRtAmpRecpr : Outport  Port=5
  MotAg5SinRtOffs : Outport  Port=6
  MotCtrlMotAgMeasTi : Outport  Port=7
  MotCtrlMotAg5Mecl : Outport  Port=8
  MotCtrlMotAg5RawMecl : Outport  Port=9
  MotAg5EolPrmRead : Outport  Port=10
  MotAg5EolPrmWr : Outport  Port=11

== system Ford_T3T6_ArchCnctnDigrm/Monitor System/Measured Signals/MotorAngle/ES243A_MotAg6Meas1 ==
  MotAg6Cos : Inport
  MotAg6CosAdcFaild : Inport  Port=2
  MotAg6RawMecl : Inport  Port=3
  MotAg6Sin : Inport  Port=4
  MotAg6SinAdcFaild : Inport  Port=5
  MotVelMrf : Inport  Port=6
  MotCtrlMotAg6Cos : Inport  Port=7
  MotCtrlMotAg6CosRtAmpRecpr : Inport  Port=8
  MotCtrlMotAg6CosRtOffs : Inport  Port=9
  MotCtrlMotAg6Polarity : Inport  Port=10
  MotCtrlMotAg6Sin : Inport  Port=11
  MotCtrlMotAg6SinRtAmpRecpr : Inport  Port=12
  MotCtrlMotAg6SinRtOffs : Inport  Port=13
  CnvSnpshtData_f32 : Inport  Port=14
  CnvSnpshtData_logl : Inport  Port=15
  GetNtcQlfrSts : Inport  Port=16
  MotAg6EolPrm_GetErrorStatus : Inport  Port=17
  MotAg6EolPrm_SetRamBlockStatus : Inport  Port=18
  MotAg6StVari_GetErrorStatus : Inport  Port=19
  MotAg6StVari_SetRamBlockStatus : Inport  Port=20
  SetNtcStsAndSnpshtData : Inport  Port=21
  MotAg6CosRtAmpRecpr : Outport
  MotAg6CosRtOffs : Outport  Port=2
  MotAg6MeclQlfr : Outport  Port=3
  MotAg6MeclRollgCntr : Outport  Port=4
  MotAg6SinRtAmpRecpr : Outport  Port=5
  MotAg6SinRtOffs : Outport  Port=6
  MotCtrlMotAg6Mecl : Outport  Port=7
  MotCtrlMotAg6RawMecl : Outport  Port=8
  MotAg6EolPrmRead : Outport  Port=9
  MotAg6EolPrmWr : Outport  Port=10

== system Ford_T3T6_ArchCnctnDigrm/Monitor System/Measured Signals/MotorAngle/ES247A_MotAgCmp ==
  AssiMechPolarity : Inport
  MotAgCumvAlgndMrfRev : Inport  Port=2
  MotAgCumvInid : Inport  Port=3
  MotCtrlMotAgMecl : Inport  Port=4
  MotAgCmpMotAgBackEmf_SetRamBlockStatus : Inport  Port=5
  MotAgCumvAlgndCrf : Outport
  MotAgCumvAlgndMrf : Outport  Port=2
  MotAgCumvAlgndVld : Outport  Port=3
  MotCtrlMotAgCumvAlgndMrfRev : Outport  Port=4
  MotCtrlMotAgCumvInid : Outport  Port=5
  MotCtrlMotAgElec : Outport  Port=6
  MotAgCmpBackEmfRead : Outport  Port=7
  MotAgCmpBackEmfWr : Outport  Port=8

== system Ford_T3T6_ArchCnctnDigrm/Monitor System/Measured Signals/MotorAngle/ES248A_MotAgArbn ==
  MotCtrlMotAgAMecl : Inport
  MotCtrlMotAgAMeclQlfr : Inport  Port=2
  MotCtrlMotAgAMeclRollgCntr : Inport  Port=3
  MotCtrlMotAgBMecl : Inport  Port=4
  MotCtrlMotAgBMeclQlfr : Inport  Port=5
  MotCtrlMotAgBMeclRollgCntr : Inport  Port=6
  MotCtrlMotAgMeclCorrlnSts : Inport  Port=7
  MotCtrlMotAgMecl : Outport

== system Ford_T3T6_ArchCnctnDigrm/Monitor System/Measured Signals/MotorAngle/ES249A_MotAgCorrln ==
  MotAgAMecl : Inport
  MotAgAMeclQlfr : Inport  Port=2
  MotAgAMeclRollgCntr : Inport  Port=3
  MotAgBMecl : Inport  Port=4
  MotAgBMeclQlfr : Inport  Port=5
  MotAgBMeclRollgCntr : Inport  Port=6
  MotAgCMecl : Inport  Port=7
  MotAgCMeclQlfr : Inport  Port=8
  MotAgCMeclRollgCntr : Inport  Port=9
  FltInj_u08 : Inport  Port=10
  GetNtcQlfrSts : Inport  Port=11
  SetNtcSts : Inport  Port=12
  MotAgABErrTerm : Outport
  MotAgACErrTerm : Outport  Port=2
  MotAgBCErrTerm : Outport  Port=3
  MotAgMeclCorrlnSts : Outport  Port=4
  MotAgMeclIdptSig : Outport  Port=5

== system Ford_T3T6_ArchCnctnDigrm/Monitor System/Measured Signals/MotorAngle/ES280A_MotAgSwCal ==
  MotCtrlMfgEnaSt : Inport
  MotCtrlMotAg2Cos : Inport  Port=2
  MotCtrlMotAg2CosAdcFaild : Inport  Port=3
  MotCtrlMotAg2Sin : Inport  Port=4
  MotCtrlMotAg2SinAdcFaild : Inport  Port=5
  MotCtrlMotAg5Cos : Inport  Port=6
  MotCtrlMotAg5CosAdcFaild : Inport  Port=7
  MotCtrlMotAg5Sin : Inport  Port=8
  MotCtrlMotAg5SinAdcFaild : Inport  Port=9
  MotCtrlMotAg6Cos : Inport  Port=10
  MotCtrlMotAg6CosAdcFaild : Inport  Port=11
  MotCtrlMotAg6Sin : Inport  Port=12
  MotCtrlMotAg6SinAdcFaild : Inport  Port=13
  MotCtrlVehSpd : Inport  Port=14
  SwCalStsCallBack : Inport  Port=15
  MotCtrlSwCalEna : Outport
  MotCtrlSwCalModlnIdx : Outport  Port=2
  MotCtrlSwCalPosnIdx : Outport  Port=3
  SwCalGetPrm : Outport  Port=4
  SwCalSetPrm : Outport  Port=5
  SwCalStop : Outport  Port=6
  SwCalStrt : Outport  Port=7

== system Ford_T3T6_ArchCnctnDigrm/Monitor System/Measured Signals/MotorCurrent/ES200B_CurrMeas ==
  BrdgVltg : Inport
  DiagcStsIvtr1Inactv : Inport  Port=2
  MotCurrAdcVlyA : Inport  Port=3
  MotCurrAdcVlyB : Inport  Port=4
  MotCurrAdcVlyC : Inport  Port=5
  MotVelMrf : Inport  Port=6
  Ntc5DErrCnt : Inport  Port=7
  StrtUpSt : Inport  Port=8
  SysSt : Inport  Port=9
  VehSpd : Inport  Port=10
  VehSpdVld : Inport  Port=11
  MotCtrlBrdgVltg : Inport  Port=12
  MotCtrlCurrMeasWrmIninTestCmpl : Inport  Port=13
  MotCtrlDiagcStsIvtr1Inactv : Inport  Port=14
  MotCtrlEcuTFild : Inport  Port=15
  MotCtrlMotAgElec : Inport  Port=16
  MotCtrlMotCurrAdcVlyA : Inport  Port=17
  MotCtrlMotCurrAdcVlyAAdcFaild : Inport  Port=18
  MotCtrlMotCurrAdcVlyB : Inport  Port=19
  MotCtrlMotCurrAdcVlyBAdcFaild : Inport  Port=20
  MotCtrlMotCurrAdcVlyC : Inport  Port=21
  MotCtrlMotCurrAdcVlyCAdcFaild : Inport  Port=22
  MotCtrlMotElecMeclPolarity : Inport  Port=23
  MotCtrlMotVelMrf : Inport  Port=24
  MotCtrlPhaOnTiA : Inport  Port=25
  MotCtrlPhaOnTiB : Inport  Port=26
  MotCtrlPhaOnTiC : Inport  Port=27
  MotCtrlPwmPerd : Inport  Port=28
  MotCtrlSysSt : Inport  Port=29
  CurrMeasEolGainCalSetABC_GetErrorStatus : Inport  Port=30
  CurrMeasEolGainCalSetABC_SetRamBlockStatus : Inport  Port=31
  CurrMeasEolOffsCalSetABC_GetErrorStatus : Inport  Port=32
  CurrMeasEolOffsCalSetABC_SetRamBlockStatus : Inport  Port=33
  FltInj_f32 : Inport  Port=34
  FltInj_u08 : Inport  Port=35
  GetNtcQlfrSts : Inport  Port=36
  SetNtcSts : Inport  Port=37
  CurrMeasWrmIninTestCmpl : Outport
  MotCurrEolCalSt : Outport  Port=2
  MotCurrQlfr1 : Outport  Port=3
  MotCtrlCurrMeasMotAgCorrd : Outport  Port=4
  MotCtrlMotCurrCorrdA : Outport  Port=5
  MotCtrlMotCurrCorrdB : Outport  Port=6
  MotCtrlMotCurrCorrdC : Outport  Port=7
  MotCtrlMotCurrRollgCntr1 : Outport  Port=8
  MotCtrlNtc5DErrCnt : Outport  Port=9
  CurrMeasEolGainReq : Outport  Port=10
  CurrMeasEolGainStsReq : Outport  Port=11
  CurrMeasEolOffsReq : Outport  Port=12
  CurrMeasEolOffsStsReq : Outport  Port=13
  CurrMeasGainReadReqSngIvtr : Outport  Port=14
  CurrMeasGainWrReqSngIvtr : Outport  Port=15
  CurrMeasOffsReadReqSngIvtr : Outport  Port=16
  CurrMeasOffsWrReqSngIvtr : Outport  Port=17

== system Ford_T3T6_ArchCnctnDigrm/Monitor System/Measured Signals/MotorCurrent/ES208A_CurrMeasArbn ==
  MotCtrlCurrMeasCorrlnSts : Inport
  MotCtrlCurrMeasMotAgCorrd : Inport  Port=2
  MotCtrlMotCurrCorrdA : Inport  Port=3
  MotCtrlMotCurrCorrdB : Inport  Port=4
  MotCtrlMotCurrCorrdC : Inport  Port=5
  MotCtrlMotCurrCorrdD : Inport  Port=6
  MotCtrlMotCurrCorrdE : Inport  Port=7
  MotCtrlMotCurrCorrdF : Inport  Port=8
  MotCtrlMotCurrQlfr1 : Inport  Port=9
  MotCtrlMotCurrQlfr2 : Inport  Port=10
  MotCtrlMotCurrRollgCntr1 : Inport  Port=11
  MotCtrlMotCurrRollgCntr2 : Inport  Port=12
  MotCtrlMotElecMeclPolarity : Inport  Port=13
  MotCtrlMotCurrDax : Outport
  MotCtrlMotCurrQax : Outport  Port=2

== system Ford_T3T6_ArchCnctnDigrm/Monitor System/Measured Signals/MotorCurrent/ES209B_CurrMeasCorrln ==
  DiagcStsIvtr1Inactv : Inport
  MotCurrCorrdA : Inport  Port=2
  MotCurrCorrdB : Inport  Port=3
  MotCurrCorrdC : Inport  Port=4
  MotCurrEolCalSt : Inport  Port=5
  MotCurrQlfr1 : Inport  Port=6
  MotCurrRollgCntr1 : Inport  Port=7
  SysSt : Inport  Port=8
  FltInj_u08 : Inport  Port=9
  GetNtcQlfrSts : Inport  Port=10
  SetNtcSts : Inport  Port=11
  CurrMeasCorrlnSts : Outport
  CurrMeasIdptSig : Outport  Port=2
  CurrMotSumABC : Outport  Port=3

== system Ford_T3T6_ArchCnctnDigrm/Monitor System/Measured Signals/ProcessHandwheelTorqueSignal/CM660A_HwTq1Meas ==
  HwTq1Polarity : Inport
  GetNtcQlfrSts : Inport  Port=2
  GetRefTmr1MicroSec32bit : Inport  Port=3
  GetTiSpan1MicroSec32bit : Inport  Port=4
  HwTq1Offs_SetRamBlockStatus : Inport  Port=5
  IoHwAb_SetFctPrphlHwTq1 : Inport  Port=6
  SetNtcSts : Inport  Port=7
  HwTq1 : Outport
  HwTq1Qlfr : Outport  Port=2
  HwTq1RollgCntr : Outport  Port=3
  RackLimrCcwEotSig1 : Outport  Port=4
  RackLimrCwEotSig1 : Outport  Port=5
  RackLimrEotSig1Avl : Outport  Port=6
  HwTq1MeasHwTq1AutTrim : Outport  Port=7
  HwTq1MeasHwTq1ClrTrim : Outport  Port=8
  HwTq1MeasHwTq1ReadTrim : Outport  Port=9
  HwTq1MeasHwTq1TrimPrfmdSts : Outport  Port=10
  HwTq1MeasHwTq1WrTrim : Outport  Port=11
  HwTq1MeasTrigStrt : Outport  Port=12

== system Ford_T3T6_ArchCnctnDigrm/Monitor System/Measured Signals/ProcessHandwheelTorqueSignal/CM690D_HwTq8Meas ==
  HwTq8Polarity : Inport
  CnvSnpshtData_u08 : Inport  Port=2
  FltInj_f32 : Inport  Port=3
  FltInj_u08 : Inport  Port=4
  GetNtcQlfrSts : Inport  Port=5
  GetRefTmr1MicroSec32bit : Inport  Port=6
  GetTiSpan1MicroSec32bit : Inport  Port=7
  HwTq8Offs_SetRamBlockStatus : Inport  Port=8
  IoHwAb_SetFctPrphlHwTq8 : Inport  Port=9
  SetNtcStsAndSnpshtData : Inport  Port=10
  HwTq8 : Outport
  HwTq8Qlfr : Outport  Port=2
  HwTq8RollgCntr : Outport  Port=3
  RackLimrCcwEotSig8 : Outport  Port=4
  RackLimrCwEotSig8 : Outport  Port=5
  RackLimrEotSig8Avl : Outport  Port=6
  HwTq8AutTrim : Outport  Port=7
  HwTq8ClrTrim : Outport  Port=8
  HwTq8ReadTrim : Outport  Port=9
  HwTq8TrigStrt : Outport  Port=10
  HwTq8TrimPrfmdSts : Outport  Port=11
  HwTq8WrTrim : Outport  Port=12

== system Ford_T3T6_ArchCnctnDigrm/Monitor System/Measured Signals/ProcessHandwheelTorqueSignal/ES224A_HwTq9Meas ==
  HwTq9Polarity : Inport
  GetNtcQlfrSts : Inport  Port=2
  GtmGetSent0Data : Inport  Port=3
  HwTq9Offs_GetErrorStatus : Inport  Port=4
  HwTq9Offs_SetRamBlockStatus : Inport  Port=5
  SetNtcSts : Inport  Port=6
  SetNtcStsAndSnpshtData : Inport  Port=7
  HwTq9 : Outport
  HwTq9Qlfr : Outport  Port=2
  HwTq9RollgCntr : Outport  Port=3
  HwTq9MeasHwTq9AutTrim : Outport  Port=4
  HwTq9MeasHwTq9ClrTrim : Outport  Port=5
  HwTq9MeasHwTq9ReadTrim : Outport  Port=6
  HwTq9MeasHwTq9TrimPrfmdSts : Outport  Port=7
  HwTq9MeasHwTq9WrTrim : Outport  Port=8

== system Ford_T3T6_ArchCnctnDigrm/Monitor System/Measured Signals/ProcessHandwheelTorqueSignal/ES225A_HwTq10Meas ==
  HwTq10Polarity : Inport
  GetNtcQlfrSts : Inport  Port=2
  GtmGetSent1Data : Inport  Port=3
  HwTq10Offs_GetErrorStatus : Inport  Port=4
  HwTq10Offs_SetRamBlockStatus : Inport  Port=5
  SetNtcSts : Inport  Port=6
  SetNtcStsAndSnpshtData : Inport  Port=7
  HwTq10 : Outport
  HwTq10Qlfr : Outport  Port=2
  HwTq10RollgCntr : Outport  Port=3
  HwTq10MeasHwTq10AutTrim : Outport  Port=4
  HwTq10MeasHwTq10ClrTrim : Outport  Port=5
  HwTq10MeasHwTq10ReadTrim : Outport  Port=6
  HwTq10MeasHwTq10TrimPrfmdSts : Outport  Port=7
  HwTq10MeasHwTq10WrTrim : Outport  Port=8

== system Ford_T3T6_ArchCnctnDigrm/Monitor System/Measured Signals/ProcessHandwheelTorqueSignal/ES228C_HwTqArbn ==
  HwTqA : Inport
  HwTqAQlfr : Inport  Port=2
  HwTqARollgCntr : Inport  Port=3
  HwTqB : Inport  Port=4
  HwTqBQlfr : Inport  Port=5
  HwTqBRollgCntr : Inport  Port=6
  HwTqC : Inport  Port=7
  HwTqCQlfr : Inport  Port=8
  HwTqCRollgCntr : Inport  Port=9
  HwTqCorrlnSts : Inport  Port=10
  HwTqD : Inport  Port=11
  HwTqDQlfr : Inport  Port=12
  HwTqDRollgCntr : Inport  Port=13
  FltInj_f32 : Inport  Port=14
  HwTq : Outport
